simulink model "TC"  (R2026a)
settings: Solver=VariableStepAuto
values from neighbouring files (symbols this model uses):
  Kp = 200    [params.m]    (also in tc_control.m = P.Kp0*sched)
undefined symbols (not defined in the file or in its folder): baseTorque, Error, maxTorque, minTorque
settings Model: Creator=jacks  LastModifiedBy=jacks

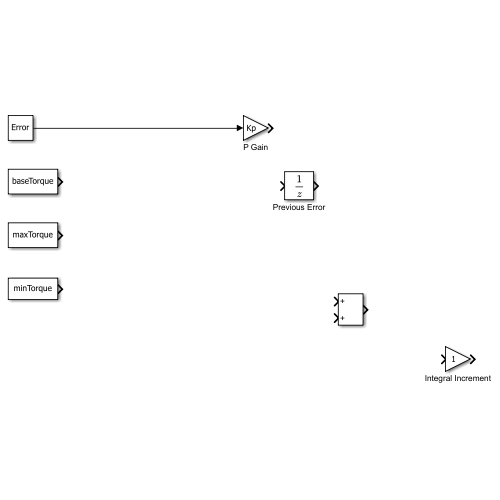
[thumbnail: Simulink's stored preview of the top-level diagram]
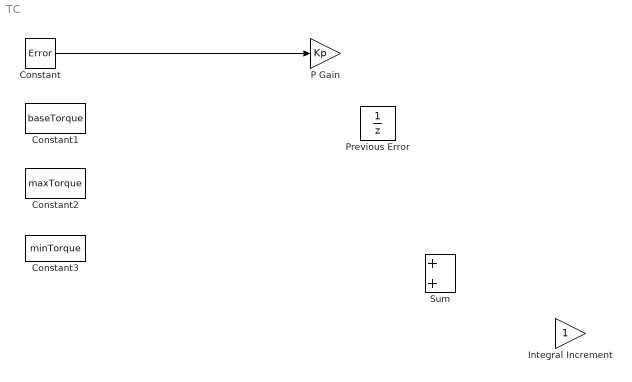
== system TC ==
  Constant : Constant  Value=Error
  Constant1 : Constant  Value=baseTorque
  Constant2 : Constant  Value=maxTorque
  Constant3 : Constant  Value=minTorque
  Integral Increment : Gain
  P Gain : Gain  Gain=Kp
  Previous Error : UnitDelay  SampleTime=-1
  Sum : Sum
  wires:
  Constant/1 -> P Gain/1
